simulink model "Model03_TestEKF"  (R2022a)
settings: Solver=FixedStepAuto  StartTime=0.0  StopTime=T1  FixedStep=Ts  RelTol=1e-3
values from neighbouring files (symbols this model uses):
  Ad = Ac*Ts+eye(2)    [KalmanFilter.m]    (also in ParaEstimation.m = Ac*Ts+eye(3); Sim01_KalmanFilter.m; Sim02_DisturbEst.m = Ac*Ts+eye(4); Sim02_ParaEstimation.m = Ac*Ts+eye(3))
  Bd = Bc*Ts    [KalmanFilter.m]    (also in ParaEstimation.m; Sim01_KalmanFilter.m; Sim02_DisturbEst.m; Sim02_ParaEstimation.m)
  C = [1 0]    [Sim03_ExtendedKF.m]
  Cd = Cc    [KalmanFilter.m]    (also in ParaEstimation.m; Sim01_KalmanFilter.m; Sim02_DisturbEst.m; Sim02_ParaEstimation.m)
  g = 9.8    [Sim03_ExtendedKF.m]
  L = 1.75    [Sim03_ExtendedKF.m]
  Q = 1e-3    (= 0.001)    [KalmanFilter.m]    (also in ParaEstimation.m = diag([0 0 Fn]); Sim01_KalmanFilter.m; Sim02_DisturbEst.m = diag([0 0 Fn 0]); Sim02_ParaEstimation.m = diag([0 0 Fn]))
  R = 1e-3    (= 0.001)    [KalmanFilter.m]    (also in ParaEstimation.m; Sim01_KalmanFilter.m; Sim02_DisturbEst.m; Sim02_ParaEstimation.m)
  Ts = 1e-3    (= 0.001)    [KalmanFilter.m]    (also in ParaEstimation.m; Sim01_KalmanFilter.m; Sim02_DisturbEst.m; Sim02_ParaEstimation.m)
  x0 = 1    [ParaEstimation.m]    (also in Sim02_DisturbEst.m; Sim02_ParaEstimation.m; Sim03_ExtendedKF.m = [1 0]')
  xk0 = [0 0]'    [Sim03_ExtendedKF.m]
libraries: simulink x2
settings Model: Creator=xiaocy  LastModifiedBy=xiaocy
settings DataIOCC: ReturnWorkspaceOutputs=off
settings DebuggingCC: UnconnectedInputMsg=warning  UnconnectedOutputMsg=warning  UnconnectedLineMsg=warning
settings RTWCC: DLArmComputeVersion=19.05

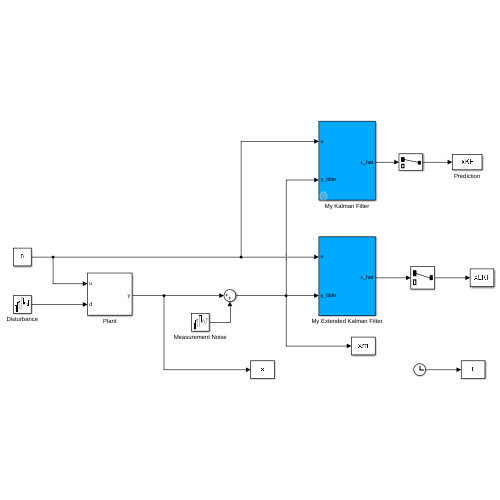
[thumbnail: Simulink's stored preview of the top-level diagram]
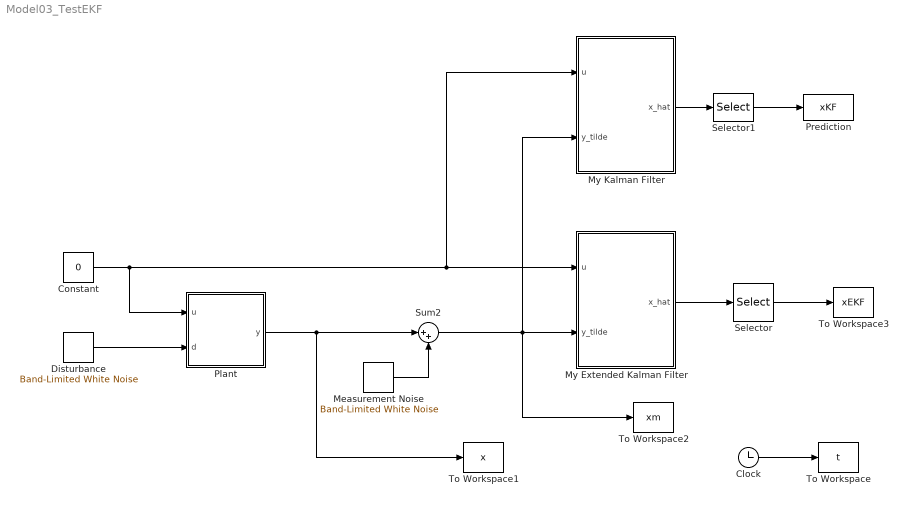
== system Model03_TestEKF ==
  Clock : Clock
  Constant : Constant  Value=0
  Disturbance : simulink/Sources/Band-Limited White Noise  Cov=Q(2,2)*Ts  Ts=Ts  seed=[23341]
  Measurement Noise : simulink/Sources/Band-Limited White Noise  Cov=R*Ts  Ts=Ts  seed=13412
  My Extended Kalman Filter : Subsystem
  My Kalman Filter : Subsystem  mask{A=Ad, B=Bd, C=Cd, Q=Q, R=R, x0=xk0, Ts=Ts}
      mask prompts: x0 "Initial state"
  Plant : Subsystem
  Prediction : ToWorkspace  VariableName=xKF  SampleTime=Ts
  Selector : Selector  InputPortWidth=2  IndexOptions=Index vector (dialog)  Indices=1  OutputSizes=1
  Selector1 : Selector  InputPortWidth=2  IndexOptions=Index vector (dialog)  Indices=1  OutputSizes=1
  Sum2 : Sum  Inputs=|++
  To Workspace : ToWorkspace  VariableName=t  SampleTime=Ts
  To Workspace1 : ToWorkspace  VariableName=x  SampleTime=Ts
  To Workspace2 : ToWorkspace  VariableName=xm  SampleTime=Ts
  To Workspace3 : ToWorkspace  VariableName=xEKF  SampleTime=Ts
  wires:
  Constant/1 -> Plant/1(u), My Kalman Filter/1(u), My Extended Kalman Filter/1(u)
  My Extended Kalman Filter/1(x_hat) -> Selector/1
  Measurement Noise/1 -> Sum2/2
  Sum2/1 -> My Kalman Filter/2(y_tilde), To Workspace2/1, My Extended Kalman Filter/2(y_tilde)
  Plant/1(y) -> To Workspace1/1, Sum2/1
  Disturbance/1 -> Plant/2(d)
  Selector/1 -> To Workspace3/1
  Clock/1 -> To Workspace/1
  My Kalman Filter/1(x_hat) -> Selector1/1
  Selector1/1 -> Prediction/1

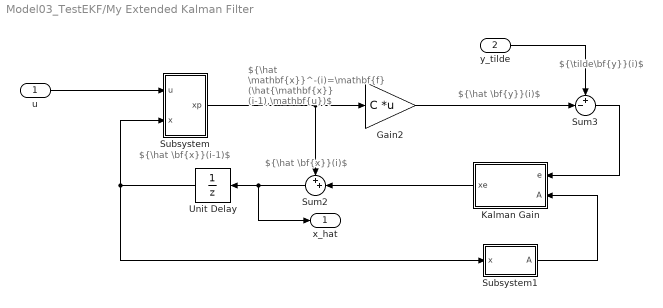
== system Model03_TestEKF/My Extended Kalman Filter ==
  note: ${\hat \bf{x}}(i)$
  note: ${\hat \bf{x}}(i-1)$
  note: ${\hat \mathbf{x}}^-(i)=\mathbf{f} (\hat{\mathbf{x}} (i-1),\mathbf{u})$
  note: ${\hat \bf{y}}(i)$
  note: ${\tilde\bf{y}}(i)$
  u : Inport
  y_tilde : Inport  Port=2
  Gain2 : Gain  Gain=C  Multiplication=Matrix(K*u)
  Kalman Gain : Subsystem
  Subsystem : Subsystem
  Subsystem1 : Subsystem
  Sum2 : Sum  Inputs=++|
  Sum3 : Sum  Inputs=+-|
  Unit Delay : UnitDelay  InitialCondition=xk0  SampleTime=Ts  HasFrameUpgradeWarning=on
  x_hat : Outport
  wires:
  Sum2/1 -> x_hat/1, Unit Delay/1
  Gain2/1 -> Sum3/2
  Sum3/1 -> Kalman Gain/1(e)
  y_tilde/1 -> Sum3/1
  Kalman Gain/1(xe) -> Sum2/2
  Subsystem/1(xp) -> Sum2/1, Gain2/1
  u/1 -> Subsystem/1(u)
  Subsystem1/1(A) -> Kalman Gain/2(A)
  Unit Delay/1 -> Subsystem1/1(x), Subsystem/2(x)

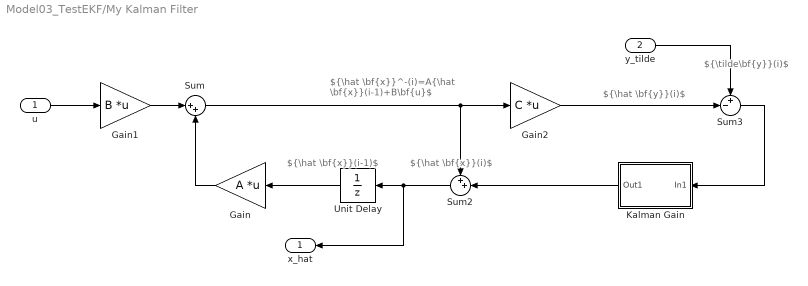
== system Model03_TestEKF/My Kalman Filter ==
  note: ${\hat \bf{x}}(i)$
  note: ${\hat \bf{x}}(i-1)$
  note: ${\hat \bf{x}}^-(i)=A{\hat \bf{x}}(i-1)+B\bf{u}$
  note: ${\hat \bf{y}}(i)$
  note: ${\tilde\bf{y}}(i)$
  u : Inport
  y_tilde : Inport  Port=2
  Gain : Gain  Gain=A  Multiplication=Matrix(K*u)
  Gain1 : Gain  Gain=B  Multiplication=Matrix(K*u)
  Gain2 : Gain  Gain=C  Multiplication=Matrix(K*u)
  Kalman Gain : Subsystem
      mask Display: disp('K')
  Sum : Sum  Inputs=|++
  Sum2 : Sum  Inputs=++|
  Sum3 : Sum  Inputs=+-|
  Unit Delay : UnitDelay  InitialCondition=x0  SampleTime=-1  HasFrameUpgradeWarning=on
  x_hat : Outport
  wires:
  Unit Delay/1 -> Gain/1
  Gain/1 -> Sum/2
  Gain1/1 -> Sum/1
  Sum/1 -> Gain2/1, Sum2/1
  Sum2/1 -> x_hat/1, Unit Delay/1
  Gain2/1 -> Sum3/2
  Sum3/1 -> Kalman Gain/1(In1)
  u/1 -> Gain1/1
  y_tilde/1 -> Sum3/1
  Kalman Gain/1(Out1) -> Sum2/2

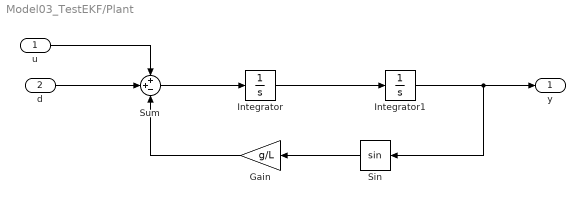
== system Model03_TestEKF/Plant ==
  u : Inport
  d : Inport  Port=2
  Gain : Gain  Gain=g/L
  Integrator : Integrator  InitialCondition=x0(2)
  Integrator1 : Integrator  InitialCondition=x0(1)
  Sin : Trigonometry
  Sum : Sum  Inputs=++-
  y : Outport
  wires:
  u/1 -> Sum/1
  Sin/1 -> Gain/1
  Gain/1 -> Sum/3
  Integrator1/1 -> y/1, Sin/1
  Sum/1 -> Integrator/1
  Integrator/1 -> Integrator1/1
  d/1 -> Sum/2

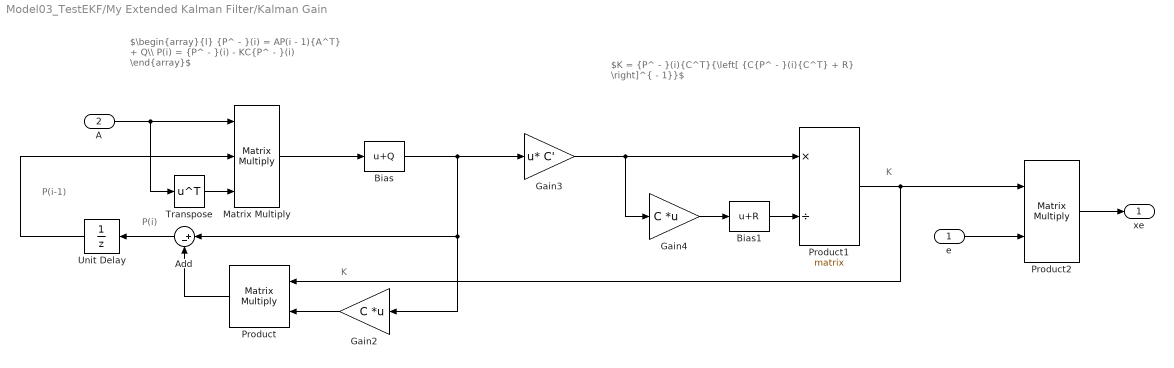
== system Model03_TestEKF/My Extended Kalman Filter/Kalman Gain ==
  note: P(i)
  note: $\begin{array}{l} {P^ - }(i) = AP(i - 1){A^T} + Q\\ P(i) = {P^ - }(i) - KC{P^ - }(i) \end{array}$
  note: $K = {P^ - }(i){C^T}{\left[ {C{P^ - }(i){C^T} + R} \right]^{ - 1}}$
  note: P(i-1)
  note: K
  note: K
  e : Inport
  A : Inport  Port=2
  Add : Sum  Inputs=|+-
  Bias : Bias  Bias=Q  SaturateOnIntegerOverflow=off
  Bias1 : Bias  Bias=R  SaturateOnIntegerOverflow=off
  Gain2 : Gain  Gain=C  Multiplication=Matrix(K*u)
  Gain3 : Gain  Gain=C'  Multiplication=Matrix(u*K)
  Gain4 : Gain  Gain=C  Multiplication=Matrix(K*u)
  Matrix Multiply : Product  Inputs=3  Multiplication=Matrix(*)
  Product : Product  Multiplication=Matrix(*)
  Product1 : Product  Inputs=*/  Multiplication=Matrix(*)
  Product2 : Product  Multiplication=Matrix(*)
  Transpose : Math  Operator=transpose
  Unit Delay : UnitDelay  SampleTime=-1  HasFrameUpgradeWarning=on
  xe : Outport
  wires:
  Unit Delay/1 -> Matrix Multiply/2
  Matrix Multiply/1 -> Bias/1
  Bias/1 -> Gain3/1, Gain2/1, Add/1
  Gain2/1 -> Product/2
  Product/1 -> Add/2
  Add/1 -> Unit Delay/1
  Gain3/1 -> Gain4/1, Product1/1
  Gain4/1 -> Bias1/1
  Bias1/1 -> Product1/2
  Product1/1 -> Product2/1, Product/1
  e/1 -> Product2/2
  Product2/1 -> xe/1
  A/1 -> Transpose/1, Matrix Multiply/1
  Transpose/1 -> Matrix Multiply/3

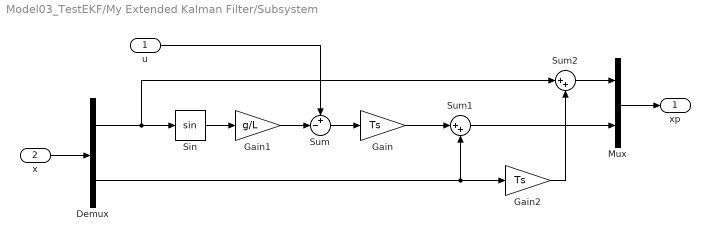
== system Model03_TestEKF/My Extended Kalman Filter/Subsystem ==
  u : Inport
  x : Inport  Port=2
  Demux : Demux  Outputs=2
  Gain : Gain  Gain=Ts
  Gain1 : Gain  Gain=g/L
  Gain2 : Gain  Gain=Ts
  Mux : Mux  Inputs=2
  Sin : Trigonometry
  Sum : Sum  Inputs=+-|
  Sum1 : Sum  Inputs=|++
  Sum2 : Sum  Inputs=|++
  xp : Outport
  wires:
  x/1 -> Demux/1
  u/1 -> Sum/1
  Demux/1 -> Sum2/1, Sin/1
  Gain1/1 -> Sum/2
  Gain/1 -> Sum1/1
  Sum/1 -> Gain/1
  Demux/2 -> Sum1/2, Gain2/1
  Sum1/1 -> Mux/2
  Sum2/1 -> Mux/1
  Gain2/1 -> Sum2/2
  Mux/1 -> xp/1
  Sin/1 -> Gain1/1

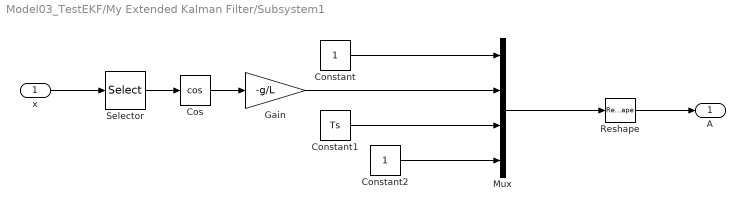
== system Model03_TestEKF/My Extended Kalman Filter/Subsystem1 ==
  x : Inport
  Constant : Constant
  Constant1 : Constant  Value=Ts
  Constant2 : Constant
  Cos : Trigonometry  Operator=cos
  Gain : Gain  Gain=-g/L
  Mux : Mux
  Reshape : Reshape  OutputDimensionality=Customize  OutputDimensions=[2,2]
  Selector : Selector  InputPortWidth=2  IndexOptions=Index vector (dialog)  Indices=1  OutputSizes=1
  A : Outport
  wires:
  Reshape/1 -> A/1
  Mux/1 -> Reshape/1
  Constant/1 -> Mux/1
  Gain/1 -> Mux/2
  Constant1/1 -> Mux/3
  Constant2/1 -> Mux/4
  x/1 -> Selector/1
  Selector/1 -> Cos/1
  Cos/1 -> Gain/1

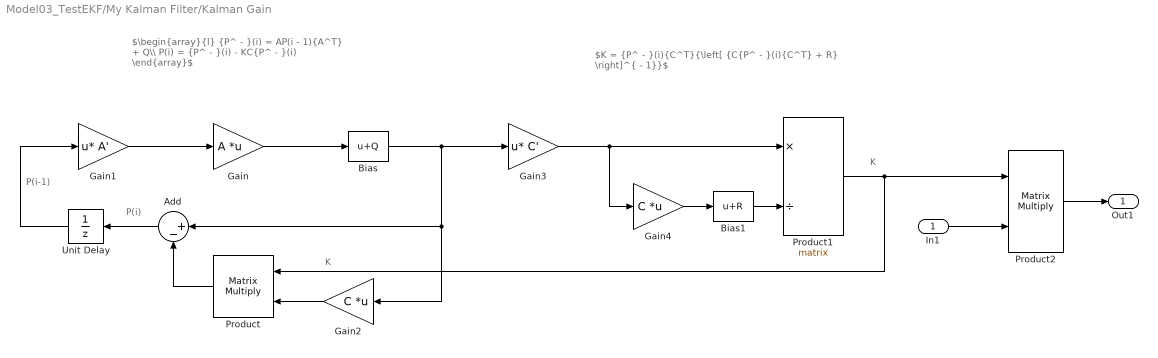
== system Model03_TestEKF/My Kalman Filter/Kalman Gain ==
  note: P(i)
  note: $\begin{array}{l} {P^ - }(i) = AP(i - 1){A^T} + Q\\ P(i) = {P^ - }(i) - KC{P^ - }(i) \end{array}$
  note: $K = {P^ - }(i){C^T}{\left[ {C{P^ - }(i){C^T} + R} \right]^{ - 1}}$
  note: P(i-1)
  note: K
  note: K
  In1 : Inport
  Add : Sum  Inputs=|+-
  Bias : Bias  Bias=Q  SaturateOnIntegerOverflow=off
  Bias1 : Bias  Bias=R  SaturateOnIntegerOverflow=off
  Gain : Gain  Gain=A  Multiplication=Matrix(K*u)
  Gain1 : Gain  Gain=A'  Multiplication=Matrix(u*K)
  Gain2 : Gain  Gain=C  Multiplication=Matrix(K*u)
  Gain3 : Gain  Gain=C'  Multiplication=Matrix(u*K)
  Gain4 : Gain  Gain=C  Multiplication=Matrix(K*u)
  Product : Product  Multiplication=Matrix(*)
  Product1 : Product  Inputs=*/  Multiplication=Matrix(*)
  Product2 : Product  Multiplication=Matrix(*)
  Unit Delay : UnitDelay  SampleTime=-1  HasFrameUpgradeWarning=on
  Out1 : Outport
  wires:
  Unit Delay/1 -> Gain1/1
  Gain1/1 -> Gain/1
  Gain/1 -> Bias/1
  Bias/1 -> Gain3/1, Gain2/1, Add/1
  Gain2/1 -> Product/2
  Product/1 -> Add/2
  Add/1 -> Unit Delay/1
  Gain3/1 -> Gain4/1, Product1/1
  Gain4/1 -> Bias1/1
  Bias1/1 -> Product1/2
  Product1/1 -> Product2/1, Product/1
  In1/1 -> Product2/2
  Product2/1 -> Out1/1
